simulink model "inverseKDynamicControl"  (R2023b)
settings: Solver=VariableStepAuto  StartTime=0.0  StopTime=10.0  RelTol=1e-3
undefined symbols (not defined in the file or in its folder): DiscIntNeverNeededParam
libraries: simulink x1
settings Model: Creator=nimro  LastModifiedBy=nimro

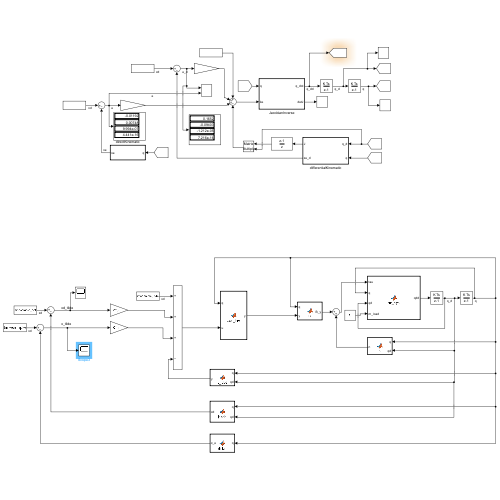
[thumbnail: Simulink's stored preview of the top-level diagram]
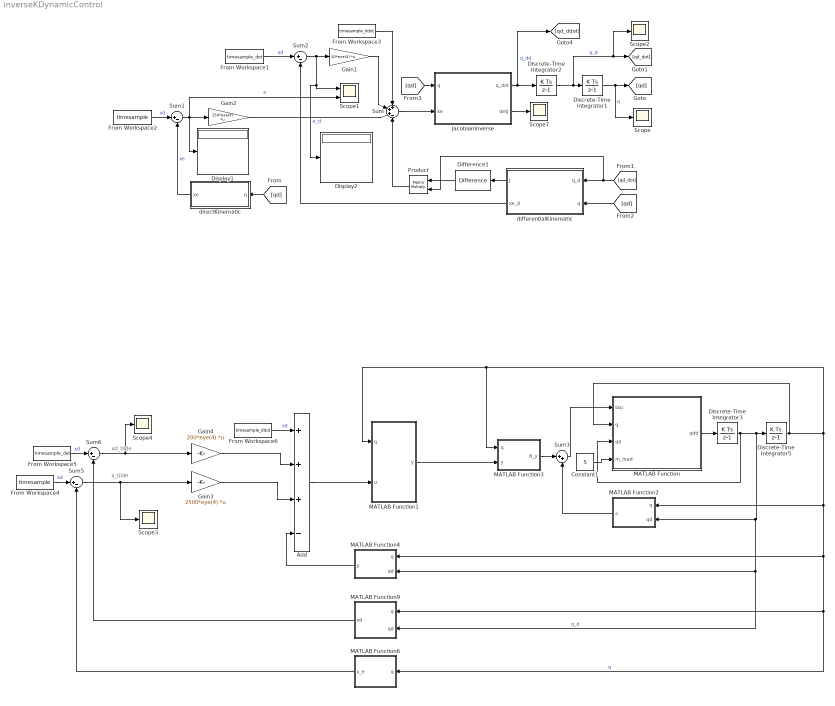
== system inverseKDynamicControl ==
  note: xd_tilde
  note: x_tilde
  Add : Sum  Inputs=+++-
  Constant1 : Constant  Value=5
  Difference1 : simulink/Discrete/Difference  ICPrevInput=0.0  OutMin=[]  OutMax=[]  OutDataType=fixdt(1, 16)  OutScaling=2^-10  DoSatur=off
  Discrete-Time Integrator1 : DiscreteIntegrator  InitialCondition=[-1.1781; 0.7851; -0.5000; 0.3930]  SampleTime=0.001  ICPrevOutput=DiscIntNeverNeededParam  ICPrevScaledInput=DiscIntNeverNeededParam
  Discrete-Time Integrator2 : DiscreteIntegrator  InitialCondition=[0; 0; 0; 0]  SampleTime=0.001  ICPrevOutput=DiscIntNeverNeededParam  ICPrevScaledInput=DiscIntNeverNeededParam
  Discrete-Time Integrator3 : DiscreteIntegrator  InitialCondition=[0; 0; 0; 0]  SampleTime=0.001  ICPrevOutput=DiscIntNeverNeededParam  ICPrevScaledInput=DiscIntNeverNeededParam
  Discrete-Time Integrator5 : DiscreteIntegrator  InitialCondition=[-1.1781; 0.7851; -0.5000; 0.3930]  SampleTime=0.001  ICPrevOutput=DiscIntNeverNeededParam  ICPrevScaledInput=DiscIntNeverNeededParam
  Display1 : Display
  Display2 : Display
  From Workspace1 : FromWorkspace  VariableName=timesample_dot
  From Workspace2 : FromWorkspace  VariableName=timesample
  From Workspace3 : FromWorkspace  VariableName=timesample_ddot
  From Workspace4 : FromWorkspace  VariableName=timesample
  From Workspace5 : FromWorkspace  VariableName=timesample_dot
  From Workspace6 : FromWorkspace  VariableName=timesample_ddot
  Gain1 : Gain  Gain=10*eye(4)  Multiplication=Matrix(K*u)
  Gain2 : Gain  Gain=150*eye(4)  Multiplication=Matrix(K*u)
  Gain3 : Gain  Gain=2500*eye(4)  Multiplication=Matrix(K*u)
  Gain4 : Gain  Gain=200*eye(4)  Multiplication=Matrix(K*u)
  JacobianInverse : MATLAB Function  TreatAsAtomicUnit=on
  MATLAB Function : MATLAB Function  TreatAsAtomicUnit=on
  MATLAB Function1 : MATLAB Function  TreatAsAtomicUnit=on
  MATLAB Function2 : MATLAB Function  TreatAsAtomicUnit=on
  MATLAB Function3 : MATLAB Function  TreatAsAtomicUnit=on
  MATLAB Function4 : MATLAB Function  TreatAsAtomicUnit=on
  MATLAB Function6 : MATLAB Function  TreatAsAtomicUnit=on
  MATLAB Function9 : MATLAB Function  TreatAsAtomicUnit=on
  Product : Product  Multiplication=Matrix(*)
  Scope{,2..4,7} (5 alike) : Scope
  Scope1 : Scope  NumInputPorts=2
  Sum : Sum  Inputs=+++-
  Sum{1..2,5..6} (4 alike) : Sum  Inputs=|+-
  Sum3 : Sum  Inputs=|++
  differentialKinematic : MATLAB Function  TreatAsAtomicUnit=on
  directKinematic : MATLAB Function  TreatAsAtomicUnit=on
  wires:
  Gain1/1 -> Sum/2
  differentialKinematic/1(J) -> Difference1/1
  [qd_dot] -> Product/2, differentialKinematic/1(q_d)
  directKinematic/1(xe) -> Sum1/2  "xe"
  From Workspace1/1 -> Sum2/1  "xd"
  [qd] -> JacobianInverse/1(q)
  Discrete-Time Integrator1/1 -> Scope/1, [qd]  "q"
  Sum1/1 -> Scope1/2, Display1/1, Gain2/1  "e"
  Difference1/1 -> Product/1
  Product/1 -> Sum/4
  Sum2/1 -> Display2/1, Scope1/1, Gain1/1  "e_d"
  JacobianInverse/2(detJ) -> Scope7/1
  From Workspace3/1 -> Sum/1
  Discrete-Time Integrator2/1 -> Scope2/1, [qd_dot], Discrete-Time Integrator1/1  "q_d"
  Gain2/1 -> Sum/3
  From Workspace2/1 -> Sum1/1  "xd"
  [qd] -> differentialKinematic/2(q)
  [qd] -> directKinematic/1(q)
  Sum/1 -> JacobianInverse/2(ke)
  differentialKinematic/2(xe_d) -> Sum2/2
  JacobianInverse/1(q_dot) -> [qd_ddot], Discrete-Time Integrator2/1  "q_dd"
  Constant1/1 -> MATLAB Function/4(m_load)
  Sum3/1 -> MATLAB Function/1(tau)
  MATLAB Function/1(qdd) -> Discrete-Time Integrator3/1
  Discrete-Time Integrator3/1 -> MATLAB Function/3(qd), MATLAB Function9/2(qd), MATLAB Function4/2(qd), MATLAB Function2/2(qd), Discrete-Time Integrator5/1  "q_d"
  Discrete-Time Integrator5/1 -> MATLAB Function/2(q), MATLAB Function1/1(q), MATLAB Function3/1(q), MATLAB Function2/1(q), MATLAB Function4/1(q), MATLAB Function6/1(q), MATLAB Function9/1(q)  "q"
  Sum6/1 -> Scope4/1, Gain4/1
  MATLAB Function9/1(xd) -> Sum6/2
  MATLAB Function4/1(y) -> Add/4
  Sum5/1 -> Scope3/1, Gain3/1
  Add/1 -> MATLAB Function1/2(u)
  MATLAB Function3/1(B_y) -> Sum3/1
  MATLAB Function1/1(y) -> MATLAB Function3/2(y)
  MATLAB Function6/1(x_e) -> Sum5/2
  MATLAB Function2/1(n) -> Sum3/2
  Gain3/1 -> Add/3
  Gain4/1 -> Add/2
  From Workspace4/1 -> Sum5/1  "xd"
  From Workspace5/1 -> Sum6/1  "xd"
  From Workspace6/1 -> Add/1  "xd"

== matlab function inverseKDynamicControl/differentialKinematic ==
  data: q_d input; J output; q input; xe_d output
function [J, xe_d] = Jacobian(q_d, q)

    % Init the SCARA manipulator parameters
    a1 = .5; a2 = .5;
    theta1 = q(1,:); theta2 = q(2,:);
    
    %% Geometric Jacobian Matrix
    J_a = [-a1*sin(theta1) - a2*sin(theta1 + theta2), - a2*sin(theta1 + theta2), 0, 0;
        a1*cos(theta1) + a2*cos(theta1 + theta2), a2*cos(theta1 + theta2), 0, 0;
        0, 0, -1, 0;
        1, 1, 0, -1;];

    % Vx = Jx1 * qd1 + Jx2 * qd2 +Jx3 * qd3;
    % Vy = Jy1 * qd1 + Jy2 * qd2 +Jy3 * qd3;
    % Vz = Jz1 * qd1 + Jz2 * qd2 +Jz3 * qd3;
    
    %J = J_a(1:3,1:3);
    J = J_a;

    %% Calculation of xe_dot
    xe_d = J * q_d;

end

== matlab function inverseKDynamicControl/directKinematic ==
  data: q input; xe output
function xe = directKinematic(q)
    
    %% Init the SCARA manipulator parameters and Joint variables
    a1 = .5; a2 = .5; d0 = 1;
    theta1 = q(1,:); theta2 = q(2,:); d3 = q(3,:); theta4 = q(4,:);

    %% Forward Kinematics link for the SCARA
    k = [a1*cos(theta1) + a2*cos(theta1 + theta2);
        a1*sin(theta1) + a2*sin(theta1 + theta2);
        d0 - d3;
        theta1 + theta2 - theta4;];

    xe = k;

end

== matlab function inverseKDynamicControl/MATLAB Function2 ==
  data: q input; n output; qd input
function n = n(q,qd)

q1 = q(1,:);
q2 = q(2,:);
q3 = q(3,:);
q4 = q(4,:);
qd1 = qd(1,:);
qd2 = qd(2,:);
qd3 = qd(3,:);
qd4 = qd(4,:);



a1 = 0.5;
a2 = 0.5;
d0 = 1;

ml1 = 20;
ml2 = 20;
ml3 = 10;
Il1 = 4;
Il2 = 4;
Il4 = 1;
Im1 = 0.01;
Im2 = 0.01;
Im3 = 0.005;
Im4 = 0.001;
l1 = 0.25;
l2 = 0.25;
kr1 = 1;
kr2 = 1;
kr3 = 50;
kr4 = 20;
Fm1 =  0.00005;
Fm2 =  0.00005;
Fm3 = 0.01;
Fm4 = 0.005;
%% calcolo p pl z
p0 = [0 ; 0 ; d0];
p1 = [a1*cos(q1) ; a1*sin(q1) ; d0];
p2 = [a1*cos(q1) + a2*cos(q1+q2) ; a1*sin(q1) + a2*sin(q1+q2) ; d0];
p3 = p2 - [0 ; 0 ; q3];
p4 = p3;
pl1 = [l1*cos(q1) ; l1*sin(q1) ; d0];
pl2 = [a1*cos(q1) + l2*cos(q1+q2) ; a1*sin(q1) + l2*sin(q1+q2) ; d0];
pl3 = p3; % ????
pl4 = p4; % ????
% pm1 = p0;
% pm2 = p1;
% pm3 = p2;
% pm4 = p3;
z0 = [0 0 1]';
z1 = [0 0 1]';
z2 = [0 0 -1]';
z3 = [0 0 -1]';
z4 = [0 0 -1]';

%% calcolo JPl JOl JOm
JP_l1 = [cross(z0,pl1-p0) zeros(3,3)];
JP_l2 = [cross(z0,pl2-p0) cross(z1,pl2-p1) zeros(3,2)];
JP_l3 = [cross(z0,pl3-p0) cross(z1,pl3-p1) z2 zeros(3,1)]; 
JP_l4 = [cross(z0,pl4-p0) cross(z1,pl4-p1) z2 cross(z3,pl4-p3)]; %m4=0
JO_l1 = [z0 zeros(3,3)];
JO_l2 = [z0 z1 zeros(3,2)];
%JO_l3 = [z0 z1 zeros(3,2)]; Il3=0
JO_l4 = [z0 z1 zeros(3,1) z3];
%JP_m1 = [zeros(4,3)]; mm1=0
%JP_m2 = [cross(z0,pm2-p0) zeros(3,3)]; mm2=0
%JP_m3 = [cross(z0,pm3-p0) cross(z1,pm3-p1) zeros(3,2)]; mm3=0
%JP_m4 = [cross(z0,pm4-p0) cross(z1,pm4-p1) cross(z2,pm3-p2) zeros(3,1)]; mm4=0
JO_m1 = JO_l1;
JO_m1(:,1) = kr1*z0;
JO_m2 = JO_l2;  
JO_m2(:,2) = kr2*z1;
JO_m3 = [z0 z1 zeros(3,2)]; 
JO_m3(:,3) = kr3*z2;
JO_m4 = JO_l4;  
JO_m4(:,4) = kr4*z3;

%% calcolo della B
B1 = ml1*(JP_l1'*JP_l1) + Il1*(JO_l1'*JO_l1) + Im1*(JO_m1'*JO_m1) ; 
B2 = ml2*(JP_l2'*JP_l2) + Il2*(JO_l2'*JO_l2) + Im2*(JO_m2'*JO_m2) ; 
B3 = ml3*(JP_l3'*JP_l3) + 0 + Im3*(JO_m3'*JO_m3) ; %Il3=0
B4 = 0 + Il4*(JO_l4'*JO_l4) + Im4*(JO_m4'*JO_m4) ; %m4=0
B = B1 + B2 + B3 + B4;

%% calcolo della g
g0 = [0 0 -9.81]';
g1 = - (ml1*g0'*JP_l1(:,1) + ml2*g0'*JP_l2(:,1) + ml3*g0'*JP_l3(:,1));
g2 = - (ml1*g0'*JP_l1(:,2) + ml2*g0'*JP_l2(:,2) + ml3*g0'*JP_l3(:,2));
g3 = - (ml1*g0'*JP_l1(:,3) + ml2*g0'*JP_l2(:,3) + ml3*g0'*JP_l3(:,3));
g4 = - (ml1*g0'*JP_l1(:,4) + ml2*g0'*JP_l2(:,4) + ml3*g0'*JP_l3(:,4));
g = [g1 g2 g3 g4]';

%% calcolo della C -> vedi file christoffel.m
C = [-a1*qd2*sin(q2)*(a2*ml3 + l2*ml2), -a1*sin(q2)*(qd1 + qd2)*(a2*ml3 + l2*ml2), 0, 0;
      a1*qd1*sin(q2)*(a2*ml3 + l2*ml2),  0, 0, 0;
      0, 0, 0, 0;
      0, 0, 0, 0];
 
%% equazione del moto
Fv=diag([kr1^2*Fm1 kr2^2*Fm2 kr3^2*Fm3 kr4^2*Fm4]);


n = C*qd + Fv*qd + g;
end

== matlab function inverseKDynamicControl/MATLAB Function1 ==
  data: q input; u input; y output
function y = Jac_inv(q,u)

q1=q(1,:);
q2=q(2,:);
q3=q(3,:);
q4=q(4,:);

a1 = 0.5;
a2 = 0.5;

    J = [-a1*sin(q1)-a2*sin(q1+q2), -a2*sin(q1+q2), 0, 0 ; a1*cos(q1)+a2*cos(q1+q2) , a2*cos(q1+q2), 0 , 0 ; 0,0,-1,0 ; 1,1,0,-1];
% 
% y = J\u;

y = inv(J)*u;
end

== matlab function inverseKDynamicControl/JacobianInverse ==
  data: q input; ke input; q_dot output; detJ output
function [q_dot, detJ] = inverseJacobian(q, ke) % q = [theta1; theta2]

    % Init the SCARA manipulator parameters
    a1 = .5; a2 = .5;

    theta1 = q(1,:); theta2 = q(2,:);
    %% Geometric Jacobian Matrix
    J = [-a1*sin(theta1) - a2*sin(theta1 + theta2), - a2*sin(theta1 + theta2), 0, 0;
        a1*cos(theta1) + a2*cos(theta1 + theta2), a2*cos(theta1 + theta2), 0, 0;
        0, 0, -1, 0;
        1, 1, 0, -1;];

    % Vx = Jx1 * qd1 + Jx2 * qd2 +Jx3 * qd3;
    % Vy = Jy1 * qd1 + Jy2 * qd2 +Jy3 * qd3;
    % Vz = Jz1 * qd1 + Jz2 * qd2 +Jz3 * qd3;
    
    %J = J(1:3,1:3);
    
    detJ = det(J);
    % Calculate the inverse of the Jacobian matrix
    J_inv = inv(J);

    % Calculate joint velocities
    q_dot = J_inv * ke;

end

== matlab function inverseKDynamicControl/MATLAB Function ==
  data: tau input; q input; qdd output; qd input; m_load input
function qdd = dir_dyn(tau,q,qd,m_load)

q1 = q(1,:);
q2 = q(2,:);
q3 = q(3,:);
q4 = q(4,:);
qd1 = qd(1,:);
qd2 = qd(2,:);

%% parametri
a1 = 0.5;
a2 = 0.5;
d0 = 1;

delta = 0.1;

ml1 = 20;
ml2 = 20;
ml3 = 10;
Il1 = 4;
Il2 = 4;
Il4 = 1;
Im1 = 0.01;
Im2 = 0.01;
Im3 = 0.005;
Im4 = 0.001;
l1 = 0.25;
l2 = 0.25;
kr1 = 1;
kr2 = 1;
kr3 = 50;
kr4 = 20;
Fm1 =  0.00005;
Fm2 =  0.00005;
Fm3 = 0.01;
Fm4 = 0.005;

% Uncertainty
% ml1 = ml1 + delta*ml1; ml2 = ml2 + delta*ml2; ml3 = ml3 + delta*ml3;
% Il1 = Il1 + delta*Il1; Il2 = Il2 + delta*Il2; Il4 = Il4 + delta*Il4;
% l1 = l1 + delta*l1; l2 = l2 + delta*l2;
% Fm1 = Fm1 + delta*Fm1;


%% calcolo p pl z
p0 = [0 ; 0 ; d0];
p1 = [a1*cos(q1) ; a1*sin(q1) ; d0];
p2 = [a1*cos(q1) + a2*cos(q1+q2) ; a1*sin(q1) + a2*sin(q1+q2) ; d0];
p3 = p2 - [0 ; 0 ; q3];
p4 = p3;
pl1 = [l1*cos(q1) ; l1*sin(q1) ; d0];
pl2 = [a1*cos(q1) + l2*cos(q1+q2) ; a1*sin(q1) + l2*sin(q1+q2) ; d0];
pl3 = p3; % ????
pl4 = p4; % 
z0 = [0 0 1]';
z1 = [0 0 1]';
z2 = [0 0 -1]';
z3 = [0 0 -1]';

%% calcolo JPl JOl JOm
JP_l1 = [cross(z0,pl1-p0) zeros(3,3)];
JP_l2 = [cross(z0,pl2-p0) cross(z1,pl2-p1) zeros(3,2)];
JP_l3 = [cross(z0,pl3-p0) cross(z1,pl3-p1) z2 zeros(3,1)]; 
JP_l4 = [cross(z0,pl4-p0) cross(z1,pl4-p1) z2 cross(z3,pl4-p3)]; %m4=mload

JO_l1 = [z0 zeros(3,3)];
JO_l2 = [z0 z1 zeros(3,2)];
%JO_l3 = [z0 z1 zeros(3,2)]; Il3=0
JO_l4 = [z0 z1 zeros(3,1) z3];

%assumo che zm1=z0, zm2=z1, zm3=-z2, zm4=z3-->si trova sul giunto
JO_m1 = JO_l1;
JO_m1(:,1) = kr1*z0;
JO_m2 = JO_l2;  
JO_m2(:,2) = kr2*z1;
JO_m3 = [z0 z1 zeros(3,2)]; 
JO_m3(:,3) = kr3*z2;
JO_m4 = JO_l4;
JO_m4(:,4) = kr4*z3;

%% Matrice d'Inerzia B (eq 7.32)
B1 = ml1*(JP_l1'*JP_l1) + Il1*(JO_l1'*JO_l1) + Im1*(JO_m1'*JO_m1) ; 
B2 = ml2*(JP_l2'*JP_l2) + Il2*(JO_l2'*JO_l2) + Im2*(JO_m2'*JO_m2) ; 
B3 = ml3*(JP_l3'*JP_l3) + 0 + Im3*(JO_m3'*JO_m3) ; %Il3=0
B4 = m_load*(JP_l4'*JP_l4) + Il4*(JO_l4'*JO_l4) + Im4*(JO_m4'*JO_m4) ; 
B = B1 + B2 + B3 + B4;

%% Contributo di gravità sull'iesimo link.(Formula 7.39)
g0 = [0 0 -9.81]';
g1 = - (ml1*g0'*JP_l1(:,1) + ml2*g0'*JP_l2(:,1) + ml3*g0'*JP_l3(:,1) + m_load*g0'*JP_l4(:,1));
g2 = - (ml1*g0'*JP_l1(:,2) + ml2*g0'*JP_l2(:,2) + ml3*g0'*JP_l3(:,2) + m_load*g0'*JP_l4(:,2));
g3 = - (ml1*g0'*JP_l1(:,3) + ml2*g0'*JP_l2(:,3) + ml3*g0'*JP_l3(:,3) + m_load*g0'*JP_l4(:,3));
g4 = - (ml1*g0'*JP_l1(:,4) + ml2*g0'*JP_l2(:,4) + ml3*g0'*JP_l3(:,4) + m_load*g0'*JP_l4(:,4));
g = [g1 g2 g3 g4]';

%% Contributo di accelerazione C
C = [-a1*qd2*sin(q2)*(a2*m_load + a2*ml3 + l2*ml2), -a1*sin(q2)*(qd1 + qd2)*(a2*m_load + a2*ml3 + l2*ml2), 0, 0;
      a1*qd1*sin(q2)*(a2*m_load + a2*ml3 + l2*ml2),  0, 0, 0;
      0, 0, 0, 0;
      0, 0, 0, 0]; 

%% Attrito viscoso al manipolatore
Fv = diag([kr1^2*Fm1 kr2^2*Fm2 kr3^2*Fm3 kr4^2*Fm4]);

%% Calcolo solo l'accelerazione dato che velox e pos si ottengono integrando
qdd = inv(B)*(tau - C*qd -Fv*qd -g);

end

== matlab function inverseKDynamicControl/MATLAB Function3 ==
  data: q input; B_y output; y input
function B_y = B(q,y)

q1 = q(1,:);
q2 = q(2,:);
q3 = q(3,:);
q4 = q(4,:);

a1 = 0.5;
a2 = 0.5;
d0 = 1;

ml1 = 20;
ml2 = 20;
ml3 = 10;
Il1 = 4;
Il2 = 4;
Il4 = 1;
Im1 = 0.01;
Im2 = 0.01;
Im3 = 0.005;
Im4 = 0.001;
l1 = 0.25;
l2 = 0.25;
kr1 = 1;
kr2 = 1;
kr3 = 50;
kr4 = 20;
Fm1 =  0.00005;
Fm2 =  0.00005;
Fm3 = 0.01;
Fm4 = 0.005;
%% calcolo p pl z
p0 = [0 ; 0 ; d0];
p1 = [a1*cos(q1) ; a1*sin(q1) ; d0];
p2 = [a1*cos(q1) + a2*cos(q1+q2) ; a1*sin(q1) + a2*sin(q1+q2) ; d0];
p3 = p2 - [0 ; 0 ; q3];
p4 = p3;
pl1 = [l1*cos(q1) ; l1*sin(q1) ; d0];
pl2 = [a1*cos(q1) + l2*cos(q1+q2) ; a1*sin(q1) + l2*sin(q1+q2) ; d0];
pl3 = p3; % ????
pl4 = p4; % ????
% pm1 = p0;
% pm2 = p1;
% pm3 = p2;
% pm4 = p3;
z0 = [0 0 1]';
z1 = [0 0 1]';
z2 = [0 0 -1]';
z3 = [0 0 -1]';
z4 = [0 0 -1]';

%% calcolo JPl JOl JOm
JP_l1 = [cross(z0,pl1-p0) zeros(3,3)];
JP_l2 = [cross(z0,pl2-p0) cross(z1,pl2-p1) zeros(3,2)];
JP_l3 = [cross(z0,pl3-p0) cross(z1,pl3-p1) z2 zeros(3,1)]; 
JP_l4 = [cross(z0,pl4-p0) cross(z1,pl4-p1) z2 cross(z3,pl4-p3)]; %m4=0
JO_l1 = [z0 zeros(3,3)];
JO_l2 = [z0 z1 zeros(3,2)];
%JO_l3 = [z0 z1 zeros(3,2)]; Il3=0
JO_l4 = [z0 z1 zeros(3,1) z3];
%JP_m1 = [zeros(4,3)]; mm1=0
%JP_m2 = [cross(z0,pm2-p0) zeros(3,3)]; mm2=0
%JP_m3 = [cross(z0,pm3-p0) cross(z1,pm3-p1) zeros(3,2)]; mm3=0
%JP_m4 = [cross(z0,pm4-p0) cross(z1,pm4-p1) cross(z2,pm3-p2) zeros(3,1)]; mm4=0
JO_m1 = JO_l1;
JO_m1(:,1) = kr1*z0;
JO_m2 = JO_l2;  
JO_m2(:,2) = kr2*z1;
JO_m3 = [z0 z1 zeros(3,2)]; 
JO_m3(:,3) = kr3*z2;
JO_m4 = JO_l4;  
JO_m4(:,4) = kr4*z3;

%% calcolo della B
B1 = ml1*(JP_l1'*JP_l1) + Il1*(JO_l1'*JO_l1) + Im1*(JO_m1'*JO_m1) ; 
B2 = ml2*(JP_l2'*JP_l2) + Il2*(JO_l2'*JO_l2) + Im2*(JO_m2'*JO_m2) ; 
B3 = ml3*(JP_l3'*JP_l3) + 0 + Im3*(JO_m3'*JO_m3) ; %Il3=0
B4 = 0 + Il4*(JO_l4'*JO_l4) + Im4*(JO_m4'*JO_m4) ; %m4=0
B = B1 + B2 + B3 + B4;
B_y = B*y;
end

== matlab function inverseKDynamicControl/MATLAB Function4 ==
  data: q input; y output; qd input
function y = J_dot(q,qd)

q1=q(1,:);
q2=q(2,:);
q3=q(3,:);
q4=q(4,:);

qd1=qd(1,:); 
qd2=qd(2,:);
qd3=qd(3,:); 
qd4=qd(4,:); 

a1 = 0.5;
a2 = 0.5;

Jdot = [-a1*cos(q1)*qd1- a2*cos(q1+q2)*(qd1+qd2) ,-a2*cos(q1+q2)*(qd1+qd2), 0 , 0 ;
        -a1*sin(q1)*qd1- a2*sin(q1+q2)*(qd1+qd2) ,-a2*sin(q1+q2)*(qd1+qd2), 0 , 0 ;
        zeros(2,4)];

y = Jdot*qd;
end

== matlab function inverseKDynamicControl/MATLAB Function6 ==
  data: q input; x_e output
function x_e = dirkin(q)
q1 = q(1,:);
q2 = q(2,:);
q3 = q(3,:);
q4 = q(4,:);

a1 = 0.5;
a2 = 0.5;
d0 = 1;
x_e = zeros(4,1);
x_e = [a1*cos(q1)+a2*cos(q1+q2) ; 
        a1*sin(q1)+a2*sin(q1+q2) ;
        d0 - q3;
        q1 + q2 - q4 ];

end

== matlab function inverseKDynamicControl/MATLAB Function9 ==
  data: q input; qd input; xd output
function xd = jacob(q,qd)

q1=q(1,:);
q2=q(2,:);
q3=q(3,:);
q4=q(4,:);

a1 = 0.5;
a2 = 0.5;

    J = [-a1*sin(q1)-a2*sin(q1+q2), -a2*sin(q1+q2), 0, 0 ; a1*cos(q1)+a2*cos(q1+q2) , a2*cos(q1+q2), 0 , 0 ; 0,0,-1,0 ; 1,1,0,-1];

xd = J*qd;
